simulink library "NeuroMuscularLibrary"  (R2019b)
settings: Solver=ode45  StartTime=0.0  StopTime=10.0  RelTol=1e-3  EnableMultiTasking=on
values from neighbouring files (symbols this model uses):
  a_18_19 = 116    [Prosthesis3R60Params.m]
  a_18_21 = 34    [Prosthesis3R60Params.m]
  a_2_3 = 18    [Prosthesis3R60Params.m]
  angle_offset = 0    [Prosthesis3R60Params.m]
  ankle_height = 0.08    [BodyMechParams.m]
  c = 0.05    [BodyMechParams.m]
  c_jointstop = 0.3 / (pi/180)    (= 17.1887338539)    [BodyMechParams.m]
  c_stance_comp_a0 = 885.0653    [Prosthesis3R60Params.m]
  c_stance_comp_a1 = 2.1443    [Prosthesis3R60Params.m]
  cg14 = 1/2*L14    (= 0.0475)    [Prosthesis3R60Params.m]
  cg25 = (5.45/11.05)*L25    (= 0.0379527149321)    [Prosthesis3R60Params.m]
  cg3 = (3.6/10.4)*L3    (= 0.0306346153846)    [Prosthesis3R60Params.m]
  d_fBall = 0.1    [BodyMechParams.m]
  d_fHeel = 0.05    [BodyMechParams.m]
  deltaLegAngleThr = 8*pi/180    (= 0.13962634016)    [CMGParams.m]
  DeltaThRef = 2e-3    (= 0.002)    [BodyMechParams.m]
  dt_visual = 0.001    [Prosthesis3R60Params.m]
  eref = 0.04    [BodyMechParams.m]
  Fmax = 4000    [MuscleEnergyTest.m]
  FmaxGLU = 1500    [BodyMechParams.m]
  footBallToAnkleDist = 0.16    [BodyMechParams.m]
  footBallToCenterDist = footLength/2    (= 0.1)    [BodyMechParams.m]
  footBallToHeelDist = footLength    (= 0.2)    [BodyMechParams.m]
  footCenterToCGDist = 0.14 - footBallToCenterDist    (= 0.04)    [BodyMechParams.m]
  footInertia = 0.005    [BodyMechParams.m]
  footLength = 0.2    [BodyMechParams.m]
  footMass = 1.25    [BodyMechParams.m]
  FT = 20    [MuscleEnergyTest.m]
  FT_GLU = 47.6    [BodyMechParams.m]
  g = 9.80665    [BodyMechParams.m]
  groundTheta = [atan(diff(groundZ)./diff(groundX)), 0]    [generateGround.m]
  groundZ = groundZ * stepSize/(largestStep+eps)    [generateGround.m]
  hatCenterToCGDist = 0.35 - hatHipToCenterDistLen    (= -0.05)    [BodyMechParams.m]
  hatHipToCenterDistLen = hatLength/2    (= 0.4)    [BodyMechParams.m]
  hatInertia = 3    [BodyMechParams.m]
  hatLeftHipToCenterDistWidth = .15    (= 0.15)    [BodyMechParams.m]
  hatLength = 0.8    [BodyMechParams.m]
  hatMass = 53.5    [BodyMechParams.m]
  hatThickness = 0.2    [BodyMechParams.m]
  hatWidth = 0.4    [BodyMechParams.m]
  J1011 = (4130)*1e-9    (= 4.13e-06)    [Prosthesis3R60Params.m]
  J1415 = (1.18*1e5)*1e-9    (= 0.000118)    [Prosthesis3R60Params.m]
  J18192021 = (6.86*1e4)*1e-9    (= 6.86e-05)    [Prosthesis3R60Params.m]
  J2526 = (3.59*1e4)*1e-9    (= 3.59e-05)    [Prosthesis3R60Params.m]
  J3467 = (25.96*1e4)*1e-9    (= 0.0002596)    [Prosthesis3R60Params.m]
  K = 5    [BodyMechParams.m]
  k_gn = k_gn/2    (= 39226.6)    [BodyMechParams.m]
  k_gt = k_gt/2    (= 39226.6)    [BodyMechParams.m]
  k_pressure = hatMass * g / DeltaThRef    (= 262327.8875)    [BodyMechParams.m]
  k_stance = 130000    [Prosthesis3R60Params.m]
  k_swing = 18750    [Prosthesis3R60Params.m]
  L0_stance = 0.08925    [Prosthesis3R60Params.m]
  L0_swing = 0.0896    [Prosthesis3R60Params.m]
  L10 = 7.9*1e-3    (= 0.0079)    [Prosthesis3R60Params.m]
  L11 = 3.3*1e-3    (= 0.0033)    [Prosthesis3R60Params.m]
  L14 = 95*1e-3    (= 0.095)    [Prosthesis3R60Params.m]
  L15 = 8.2*1e-3    (= 0.0082)    [Prosthesis3R60Params.m]
  L18 = 25.1*1e-3    (= 0.0251)    [Prosthesis3R60Params.m]
  L19 = 17.7*1e-3    (= 0.0177)    [Prosthesis3R60Params.m]
  L20 = 26*1e-3    (= 0.026)    [Prosthesis3R60Params.m]
  L21 = 1.7*1e-3    (= 0.0017)    [Prosthesis3R60Params.m]
  L25 = 76.95*1e-3    (= 0.07695)    [Prosthesis3R60Params.m]
  L26 = 2.8*1e-3    (= 0.0028)    [Prosthesis3R60Params.m]
  L3 = 88.5*1e-3    (= 0.0885)    [Prosthesis3R60Params.m]
  L4 = 1.7*1e-3    (= 0.0017)    [Prosthesis3R60Params.m]
  L6 = 40.25*1e-3    (= 0.04025)    [Prosthesis3R60Params.m]
  L7 = 14.9*1e-3    (= 0.0149)    [Prosthesis3R60Params.m]
  leg_l = [(thighLength - ankle_height/2) (shankLength - ankle_height/2)]    [BodyMechParams.m]
  legAngleSpeedMax = 10    [CMGParams.m]
  lopt = 0.055    [MuscleEnergyTest.m]
  loptBFSH = 0.12    [BodyMechParams.m]
  loptGAS = 0.05    [BodyMechParams.m]
  loptGLU = 0.11    [BodyMechParams.m]
  loptHAB = 0.09    [BodyMechParams.m]
  loptHAD = 0.10    (= 0.1)    [BodyMechParams.m]
  loptHAM = 0.10    (= 0.1)    [BodyMechParams.m]
  loptHFL = 0.11    [BodyMechParams.m]
  loptRF = 0.08    [BodyMechParams.m]
  loptSOL = 0.04    [BodyMechParams.m]
  loptTA = 0.06    [BodyMechParams.m]
  loptVAS = 0.08    [BodyMechParams.m]
  lslack = 0.245    [MuscleEnergyTest.m]
  lslackBFSH = 0.10    (= 0.1)    [BodyMechParams.m]
  lslackGAS = 0.40    (= 0.4)    [BodyMechParams.m]
  lslackGLU = 0.13    [BodyMechParams.m]
  lslackHAB = 0.07    [BodyMechParams.m]
  lslackHAD = 0.18    [BodyMechParams.m]
  lslackHAM = 0.31    [BodyMechParams.m]
  lslackHFL = 0.10    (= 0.1)    [BodyMechParams.m]
  lslackRF = 0.35    [BodyMechParams.m]
  lslackSOL = 0.26    [BodyMechParams.m]
  lslackTA = 0.24    [BodyMechParams.m]
  lslackVAS = 0.23    [BodyMechParams.m]
  m1011 = 49.5*1e-3    (= 0.0495)    [Prosthesis3R60Params.m]
  m1415 = 123.8*1e-3    (= 0.1238)    [Prosthesis3R60Params.m]
  m18192021 = 196.6*1e-3    (= 0.1966)    [Prosthesis3R60Params.m]
  m2526 = 58.3*1e-3    (= 0.0583)    [Prosthesis3R60Params.m]
  m3467 = 253.3*1e-3    (= 0.2533)    [Prosthesis3R60Params.m]
  mu_slide = 0.8    [BodyMechParams.m]
  mu_stick = 0.9    [BodyMechParams.m]
  N = 1.5    [BodyMechParams.m]    (also in cmaes.m = size(x,1); mergeCompareEnergyCosts.m = {S.name})
  phiKneeUpLimit = 5*pi/180    (= 0.0872664625997)    [BodyMechParams.m]
  phimaxGASa = (100-90)*pi/180    (= 0.174532925199)    [BodyMechParams.m]
  phimaxGASk = (180-140)*pi/180    (= 0.698131700798)    [BodyMechParams.m]
  phimaxRFk = (180-165)*pi/180    (= 0.261799387799)    [BodyMechParams.m]
  phimaxSOL = (100-90)*pi/180    (= 0.174532925199)    [BodyMechParams.m]
  phimaxTA = (80-90)*pi/180    (= -0.174532925199)    [BodyMechParams.m]
  phimaxVAS = (180-165)*pi/180    (= 0.261799387799)    [BodyMechParams.m]
  phirefBFSH = (180-160)*pi/180    (= 0.349065850399)    [BodyMechParams.m]
  phirefGASa = (80-90)*pi/180    (= -0.174532925199)    [BodyMechParams.m]
  phirefGASk = (180-165)*pi/180    (= 0.261799387799)    [BodyMechParams.m]
  phirefGLU = (120-180)*pi/180    (= -1.0471975512)    [BodyMechParams.m]
  phirefHAB = 10*pi/180    (= 0.174532925199)    [BodyMechParams.m]
  phirefHAD = 15*pi/180    (= 0.261799387799)    [BodyMechParams.m]
  phirefHAMh = (150-180)*pi/180    (= -0.523598775598)    [BodyMechParams.m]
  phirefHAMk = (180-180)*pi/180    (= 0)    [BodyMechParams.m]
  phirefHFL = (160-180)*pi/180    (= -0.349065850399)    [BodyMechParams.m]
  phirefRFh = (170-180)*pi/180    (= -0.174532925199)    [BodyMechParams.m]
  phirefRFk = (180-125)*pi/180    (= 0.959931088597)    [BodyMechParams.m]
  phirefSOL = (90-90)*pi/180    (= 0)    [BodyMechParams.m]
  ... (+64 more)
undefined symbols (not defined in the file or in its folder): ankleBackDriveGain, ankleCJointstop, ankleDgain, ankleFilterPID, ankleFilterSEA, ankleGearEff, ankleGearRatio, ankleIgain, ankleInitialAngle, ankleInputMass, ankleIntCoulomb, ankleIntDamping, ankleIntStatic, ankleParallelSpringDamping, ankleParallelSpringOffset, ankleParallelSpringStiffness, anklePgain, anklePlantarLimit, ankleSEADamping, ankleSEAStiffness, ankleTendonMass, ankleWMaxJointstop, D12_F, D12_S, D12_T, D12z_T, D13_F, D1G_F, D1G_HAT, D1G_S, D1G_T, D1Gy_F, DeltaS, DeltaSGLU, DeltaSHFL, dryFrictionDamping, dryFrictionStiffness, dryFrictionVelThresh, footMassp, FourBarL1, FourBarL3, GainDphiHATGLUst, GainDphiHATHABst, GainDphiHATHADst, GainDphiHATHFLst, GainFGASst, GainFGLUst, GainFHABst, GainFHAMst, GainFSOLst, GainFSOLTAst, GainFVASst, GainGAS, GainGLU, GainGLUswing, GainHAM, GainHAMHFL ... (+194)
libraries: sm_lib x332, nesl_utility x156, simulink x33, dspswit3 x30, $bdroot x19, simulink_extras x7
(part 8 of 15)

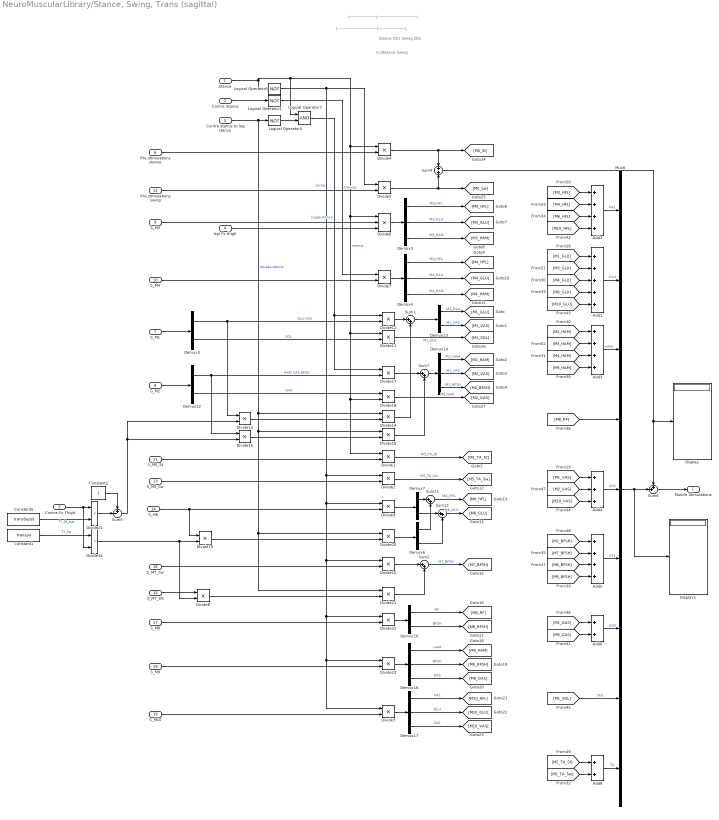
== system NeuroMuscularLibrary/Stance, Swing, Trans (sagittal) ==
  note: Stance DS1 Swing DS2
  note: FullStance Swing
  note: |------------------------------|--------------------|
  note: |--------------------|------------------------------|
  Stance : Inport
  Contra Stance : Inport  Port=2
  Contra stance to leg stance : Inport  Port=3
  Ispi Fx thigh : Inport  Port=4
  Contra Fx Thigh : Inport  Port=5
  Pre stimulations stance : Inport  Port=6
  S_M1 : Inport  Port=7
  S_M2 : Inport  Port=8
  S_M3 : Inport  Port=9
  S_M4 : Inport  Port=10
  S_M5_St : Inport  Port=11
  Pre stimulations swing : Inport  Port=12
  S_M5_Sw : Inport  Port=13
  S_M6 : Inport  Port=14
  S_M7_DS : Inport  Port=15
  S_M7_Sw : Inport  Port=16
  S_M8 : Inport  Port=17
  S_M9 : Inport  Port=18
  S_M10 : Inport  Port=19
  Add1 : Sum  Inputs=5
  Add2 : Sum  Inputs=4
  Add3 : Sum  Inputs=4
  Add4 : Sum  Inputs=3
  Add5 : Sum  Inputs=4
  Add6 : Sum  Inputs=2
  Add8 : Sum  Inputs=2
  Constant1 : Constant  Value=transsw
  Constant2 : Constant
  Constant5 : Constant  Value=transSupst
  Demux{6..7,10,13} (4 alike) : Demux  Outputs=2
  Demux12 : Demux  Outputs=[3 1]
  Demux{3..4,14,16..17} (5 alike) : Demux  Outputs=3
  Demux5 : Demux  Outputs=[2 1]
  Display : Display
  Display1 : Display
  Divide{1..5,7..24,34} (24 alike) : Product
  Divide6 : Product  Inputs=3
  Logical Operator1 : Logic  Operator=NOT  AllPortsSameDT=off  OutDataTypeStr=boolean
  Logical Operator5 : Logic  Operator=NOT  AllPortsSameDT=off  OutDataTypeStr=boolean
  Logical Operator6 : Logic  Operator=NOT  AllPortsSameDT=off  OutDataTypeStr=boolean
  Logical Operator7 : Logic  AllPortsSameDT=off  OutDataTypeStr=boolean
  Mux6 : Mux  Inputs=9
  Sum{1..2,7,11..12} (5 alike) : Sum  Inputs=|++  SaturateOnIntegerOverflow=on  InputSameDT=on  OutDataTypeStr=Inherit: Same as first input
  Sum4 : Sum  SaturateOnIntegerOverflow=on  InputSameDT=on  OutDataTypeStr=Inherit: Same as first input
  Sum5 : Sum  Inputs=+-|  SaturateOnIntegerOverflow=on  InputSameDT=on  OutDataTypeStr=Inherit: Same as first input
  Sum6 : Sum  Inputs=++|  SaturateOnIntegerOverflow=on  InputSameDT=on  OutDataTypeStr=Inherit: Same as first input
  Muscle Stimulations : Outport  OutputWhenDisabled=reset  InitialOutput=0
  wires:
  Stance/1 -> Logical Operator7/1, Divide4/1, Divide11/1, Divide18/2, Divide1/1, Divide6/1, Logical Operator6/1  "stance"
  Contra stance to leg stance/1 -> Logical Operator5/1, Divide14/1, Divide16/1, Divide20/1, Divide21/1  "double stance"
  Logical Operator5/1 -> Logical Operator7/2
  S_M4/1 -> Divide7/2
  Contra Stance/1 -> Logical Operator1/1
  Logical Operator1/1 -> Divide7/1  "Cswing"
  Constant5/1 -> Divide24/2  "Tr_St_sup"
  Divide24/1 -> Sum5/2
  Constant2/1 -> Sum5/1
  Contra Fx Thigh/1 -> Divide24/1, Divide34/2
  Demux4/1 -> [M4_HFL]  "M4_HFL"
  Add2/1 -> Mux6/1  "HFL"
  Add1/1 -> Mux6/2  "GLU"
  Demux4/2 -> [M4_GLU]  "M4_GLU"
  Add3/1 -> Mux6/3  "HAM"
  Demux4/3 -> [M4_HAM]  "M4_HAM"
  Add4/1 -> Mux6/5  "VAS"
  Add5/1 -> Mux6/6  "KFL"
  Add6/1 -> Mux6/7  "GAS"
  Add8/1 -> Mux6/9  "TA"
  Constant1/1 -> Divide34/1  "Tr_Sw"
  Divide7/1 -> Demux4/1
  Logical Operator7/1 -> Divide12/1, Divide17/1  "single stance"
  Divide34/1 -> Divide19/2, Divide8/2
  Logical Operator6/1 -> Divide5/1, Divide2/1, Divide9/1, Divide10/1, Divide3/1, Divide23/1, Divide22/1  "swing"
  Mux6/1 -> Display1/1, Sum6/2
  Sum6/1 -> Muscle Stimulations/1
  Sum4/1 -> Display/1, Sum6/1
  Pre stimulations swing/1 -> Divide5/2
  Pre stimulations stance/1 -> Divide4/2
  Divide5/1 -> [M0_Sw], Sum4/2
  Divide4/1 -> Sum4/1, [M0_St]
  S_M1/1 -> Demux5/1
  S_M2/1 -> Demux12/1
  Demux5/1 -> Divide12/2, Divide13/1  "GLU VAS"
  Demux5/2 -> Divide11/2  "SOL"
  Divide12/1 -> Sum1/1
  Divide13/1 -> Divide14/2
  Divide14/1 -> Sum1/2
  Divide16/1 -> Sum7/2
  Divide15/1 -> Divide16/2
  Sum1/1 -> Demux13/1
  Demux13/1 -> [M1_GLU]  "M1_GLU"
  Demux13/2 -> [M1_VAS]  "M1_VAS"
  Demux12/1 -> Divide17/2, Divide15/1  "HAM VAS BFSH"
  Divide17/1 -> Sum7/1
  Sum7/1 -> Demux14/1
  Demux14/1 -> [M2_HAM]  "M2_HAM"
  Demux14/2 -> [M2_VAS]  "M2_VAS"
  Demux14/3 -> [M2_BFSH]  "M2_BFSH"
  Demux12/2 -> Divide18/1  "GAS"
  Divide18/1 -> [M2_GAS]  "M2_GAS"
  S_M5_St/1 -> Divide1/2
  Divide1/1 -> [M5_TA_St]  "M5_TA_St"
  Divide11/1 -> [M1_SOL]  "M1_SOL"
  S_M3/1 -> Divide6/2
  Ispi Fx thigh/1 -> Divide6/3
  Divide6/1 -> Demux3/1
  Demux3/1 -> [M3_HFL]  "M3_HFL"
  Demux3/2 -> [M3_GLU]  "M3_GLU"
  Demux3/3 -> [M3_HAM]  "M3_HAM"
  S_M5_Sw/1 -> Divide2/2
  Divide2/1 -> [M5_TA_Sw]  "M5_TA_Sw"
  S_M6/1 -> Divide9/2, Divide19/1
  Divide9/1 -> Demux7/1
  Demux7/2 -> Sum12/1
  Divide20/1 -> Demux6/1
  Demux6/1 -> Sum11/2
  Demux6/2 -> Sum12/2
  Demux7/1 -> Sum11/1
  Divide19/1 -> Divide20/2
  Sum11/1 -> [M6_HFL]  "M6_HFL"
  Sum12/1 -> [M6_GLU]  "M6_GLU"
  Divide10/1 -> Sum2/1
  Divide21/1 -> Sum2/2
  Sum5/1 -> Divide13/2, Divide15/2
  S_M7_Sw/1 -> Divide10/2
  Divide8/1 -> Divide21/2
  S_M7_DS/1 -> Divide8/1
  Sum2/1 -> [M7_BFSH]  "M7_BFSH"
  S_M8/1 -> Divide22/2
  Divide22/1 -> Demux10/1
  S_M9/1 -> Divide23/2
  Divide23/1 -> Demux16/1
  S_M10/1 -> Divide3/2
  Divide3/1 -> Demux17/1
  Demux10/2 -> [M8_BFSH]  "BFSH"
  Demux10/1 -> [M8_RF]  "RF"
  Demux16/1 -> [M9_HAM]  "HAM"
  Demux16/2 -> [M9_BFSH]  "BFSH"
  Demux16/3 -> [M9_GAS]  "GAS"
  Demux17/1 -> [M10_HFL]  "HFL"
  Demux17/2 -> [M10_GLU]  "GLU"
  Demux17/3 -> [M10_VAS]  "VAS"
  [M1_GLU] -> Add1/1
  [M3_GLU] -> Add1/2
  [M4_GLU] -> Add1/3
  [M6_GLU] -> Add1/4
  [M10_GLU] -> Add1/5
  [M1_VAS] -> Add4/1
  [M2_HAM] -> Add3/1
  [M2_VAS] -> Add4/2
  [M2_BFSH] -> Add5/1
  [M2_GAS] -> Add6/1
  [M3_HFL] -> Add2/1
  [M3_HAM] -> Add3/2
  [M4_HFL] -> Add2/2
  [M4_HAM] -> Add3/3
  [M5_TA_St] -> Add8/1
  [M5_TA_Sw] -> Add8/2
  [M6_HFL] -> Add2/3
  [M7_BFSH] -> Add5/2
  [M9_BFSH] -> Add5/4
  [M8_BFSH] -> Add5/3
  [M8_RF] -> Mux6/4
  [M9_HAM] -> Add3/4
  [M9_GAS] -> Add6/2
  [M10_HFL] -> Add2/4
  [M10_VAS] -> Add4/3
  [M1_SOL] -> Mux6/8  "SOL"

== system NeuroMuscularLibrary/Stimulation Mixing ==
  Stance Stim : Inport
  dxThigh : Inport  Port=2
  Stance? : Inport  Port=3
  ContraLegLeading? : Inport  Port=4
  Swing Stim : Inport  Port=5
  Constant : Constant
  FB Gain1 : Gain  Gain=1/DeltaThRef  SaturateOnIntegerOverflow=on  OutDataTypeStr=Inherit: Same as input  ParamDataTypeStr=Inherit: Same as input
  Logical Operator : Logic  Operator=NOT  AllPortsSameDT=off  OutDataTypeStr=boolean
  Logical Operator1 : Logic  Operator=NOT  AllPortsSameDT=off  OutDataTypeStr=boolean
  Product{,1..3} (4 alike) : Product
  Product4 : Product  Inputs=3
  Saturation17 : Saturate  UpperLimit=1  LowerLimit=0.01  ZeroCross=off
  Saturation2 : Saturate  UpperLimit=1  LowerLimit=0  ZeroCross=off
  Sum : Sum  Inputs=+|+
  Sum1 : Sum  Inputs=-+|
  Sum3 : Sum  Inputs=+++
  stimulation : Outport  OutputWhenDisabled=reset
  wires:
  dxThigh/1 -> FB Gain1/1
  Stance Stim/1 -> Product4/1, Product/1
  FB Gain1/1 -> Saturation2/1
  Saturation2/1 -> Product/2, Sum1/1
  Swing Stim/1 -> Product3/1, Product1/2
  Constant/1 -> Sum1/2
  Sum1/1 -> Product1/1
  Product1/1 -> Sum/2
  Product/1 -> Sum/1
  Logical Operator/1 -> Product4/3
  Stance?/1 -> Logical Operator1/1, Product4/2
  Sum/1 -> Product2/1
  Product2/1 -> Sum3/2  "Mixed Stimulation"
  Sum3/1 -> Saturation17/1
  Saturation17/1 -> stimulation/1
  Product4/1 -> Sum3/1  "Stance Stimulation Only"
  Logical Operator1/1 -> Product3/2
  Product3/1 -> Sum3/3  "Swing Stimulation Only"
  ContraLegLeading?/1 -> Product2/2, Logical Operator/1

== system NeuroMuscularLibrary/Subsystem ==
  Thigh dx : Inport

== system NeuroMuscularLibrary/Swing Hip & Ankles ==
  note: Stimulation
  note: Torques
  note: Hip Torque
  note: GLU Control
  note: GAS Control
  note: TA Control
  note: VAS Control
  note: SOL Control
  note: HAM Control
  note: HFL Control
  Muscle Torques : Inport
  LceTA : Inport  Port=2
  FmHAM : Inport  Port=3
  FmGLU : Inport  Port=4
  LceHFL : Inport  Port=5
  LceHAM : Inport  Port=6
  phiANDdphiHAT : Inport  Port=7
  " 3" : Gain  Gain=GainTA
  Add3 : Sum
  Add4 : Sum  Inputs=++-+
  Add7 : Sum
  Add8 : Sum
  Constant1 : Constant  Value=PreStimGAS
  Constant2 : Constant  Value=PreStimVAS
  Constant4 : Constant  Value=PreStimTA
  Constant6 : Constant  Value=PreStimSOL
  Count Extend : dspswit3/Counter  Direction=Up  CountEvent=Rising edge  CounterSize=16 bits  MaxCount=255  InitialCount=0  Output=Count  HitValue=32  ResetInput=off  SamplesPerFrame=1  Ts=1  CntDtype=double  HitDtype=Logical
  Count Flex : dspswit3/Counter  Direction=Up  CountEvent=Rising edge  CounterSize=16 bits  MaxCount=255  InitialCount=0  Output=Count  HitValue=32  ResetInput=off  SamplesPerFrame=1  Ts=1  CntDtype=double  HitDtype=Logical
  Count Hold : dspswit3/Counter  Direction=Up  CountEvent=Rising edge  CounterSize=16 bits  MaxCount=255  InitialCount=0  Output=Count  HitValue=32  ResetInput=off  SamplesPerFrame=1  Ts=1  CntDtype=double  HitDtype=Logical
  Count Stancea : dspswit3/Counter  Direction=Up  CountEvent=Rising edge  CounterSize=16 bits  MaxCount=255  InitialCount=0  Output=Count  HitValue=32  ResetInput=off  SamplesPerFrame=1  Ts=1  CntDtype=double  HitDtype=Logical
  Count Stop : dspswit3/Counter  Direction=Up  CountEvent=Rising edge  CounterSize=16 bits  MaxCount=255  InitialCount=0  Output=Count  HitValue=32  ResetInput=off  SamplesPerFrame=1  Ts=1  CntDtype=double  HitDtype=Logical
  Demux : Demux  Outputs=3
  Demux2 : Demux  Outputs=2
  FB Gain1 : Gain  Gain=GainHAM  SaturateOnIntegerOverflow=on  OutDataTypeStr=Inherit: Same as input  ParamDataTypeStr=Inherit: Same as input
  FB Gain11 : Gain  Gain=Klean  SaturateOnIntegerOverflow=on  OutDataTypeStr=Inherit: Same as input  ParamDataTypeStr=Inherit: Same as input
  FB Gain2 : Gain  Gain=GainHFL  SaturateOnIntegerOverflow=on  OutDataTypeStr=Inherit: Same as input  ParamDataTypeStr=Inherit: Same as input
  FB Gain4 : Gain  Gain=GainHAMHFL  SaturateOnIntegerOverflow=on  OutDataTypeStr=Inherit: Same as input  ParamDataTypeStr=Inherit: Same as input
  FB Gain5 : Gain  Gain=GainGLU  SaturateOnIntegerOverflow=on  OutDataTypeStr=Inherit: Same as input  ParamDataTypeStr=Inherit: Same as input
  Multiply : Gain
  Multiply1 : Gain
  Multiply2 : Gain
  Mux1 : Mux  Inputs=7
  Mux2 : Mux  Inputs=3
  Mux3 : Mux  Inputs=5
  Mux4 : Mux  Inputs=3
  Stimulation Bias4 : Constant  Value=PreStimHFL
  Stimulation Bias5 : Constant  Value=PreStimHAM
  Stimulation Bias6 : Constant  Value=phiHATref
  Stimulation Bias8 : Constant  Value=PreStimGLU
  Sum9 : Sum  Inputs=|+-  SaturateOnIntegerOverflow=on  InputSameDT=on  OutDataTypeStr=Inherit: Same as first input
  Terminator : Terminator
  ideal ankle torque{,1..7} (8 alike) : Constant  Value=0
  Stimulation : Outport
  Swing Muscle Torques : Outport  Port=2
  Swing Ideal Torques : Outport  Port=3
  Swing State Counts : Outport  Port=4
  wires:
  Demux/2 -> Mux4/2
  Demux/3 -> Mux4/3
  Mux4/1 -> Swing Muscle Torques/1
  Constant6/1 -> Mux1/1
  Add3/1 -> Mux1/2
  Add8/1 -> Mux1/6
  Add4/1 -> Mux1/7
  Add7/1 -> Mux1/5
  ideal ankle torque3/1 -> Count Stancea/1
  ideal ankle torque6/1 -> Count Stop/1
  Count Flex/1 -> Mux3/2
  ideal ankle torque1/1 -> Mux2/2
  ideal ankle torque2/1 -> Mux2/1
  ideal ankle torque5/1 -> Count Hold/1
  Count Hold/1 -> Mux3/3
  ideal ankle torque/1 -> Mux2/3
  Mux3/1 -> Swing State Counts/1
  Count Stancea/1 -> Mux3/1
  ideal ankle torque4/1 -> Count Flex/1
  ideal ankle torque7/1 -> Count Extend/1
  Mux2/1 -> Swing Ideal Torques/1
  Count Extend/1 -> Mux3/5
  Mux1/1 -> Stimulation/1
  FmHAM/1 -> FB Gain1/1
  " 3"/1 -> Add3/2
  phiANDdphiHAT/1 -> Demux2/1
  LceHFL/1 -> FB Gain2/1
  Stimulation Bias8/1 -> Multiply/1
  Stimulation Bias5/1 -> Multiply2/1
  Constant2/1 -> Mux1/4
  Sum9/1 -> FB Gain11/1
  FB Gain5/1 -> Add8/2
  Demux/1 -> Mux4/1
  FmGLU/1 -> FB Gain5/1
  Demux2/1 -> Sum9/1  "phiHAT"
  Count Stop/1 -> Mux3/4
  LceTA/1 -> " 3"/1
  Demux2/2 -> Terminator/1  "dphiHat"
  Muscle Torques/1 -> Demux/1
  FB Gain11/1 -> Add4/4
  Stimulation Bias6/1 -> Sum9/2
  LceHAM/1 -> FB Gain4/1
  FB Gain2/1 -> Add4/2
  Stimulation Bias4/1 -> Multiply1/1
  FB Gain1/1 -> Add7/2
  FB Gain4/1 -> Add4/3
  Constant1/1 -> Mux1/3
  Multiply/1 -> Add8/1
  Multiply1/1 -> Add4/1
  Multiply2/1 -> Add7/1
  Constant4/1 -> Add3/1

== system NeuroMuscularLibrary/Swing Phase ==
  note: Stimulation
  note: SOL Control
  note: GAS Control
  note: TA Control
  note: VAS Control
  note: HAM Control
  note: GLU Control
  note: HFL Control
  note: Torques
  note: Hip Torque
  note: only ankle muscle torque
  Muscle Torques : Inport
  LceTA : Inport  Port=2
  Leg Angle : Inport  Port=3
  Leg Length : Inport  Port=4
  Stance? : Inport  Port=5
  contraStance? : Inport  Port=6
  Knee Speed : Inport  Port=7
  Target Leg Angle : Inport  Port=8
  " 1" : Gain  Gain=hipPGain
  " 2" : Gain  Gain=hipDGain
  " 3" : Gain  Gain=GainTA
  " 4" : Gain  Gain=2
  " 5" : Gain  Gain=0
  " 6" : Gain  Gain=0
  Add : Sum  Inputs=+++
  Add1 : Sum  Inputs=+-+
  Add3 : Sum
  Chart : Stateflow chart  TreatAsAtomicUnit=on
  Constant{1..3,5..7} (6 alike) : Constant  Value=0
  Constant4 : Constant  Value=PreStimTA
  Count Extend : dspswit3/Counter  Direction=Up  CountEvent=Rising edge  CounterSize=16 bits  MaxCount=255  InitialCount=0  Output=Count  HitValue=32  ResetInput=off  SamplesPerFrame=1  Ts=1  CntDtype=double  HitDtype=Logical
  Count Flex : dspswit3/Counter  Direction=Up  CountEvent=Rising edge  CounterSize=16 bits  MaxCount=255  InitialCount=0  Output=Count  HitValue=32  ResetInput=off  SamplesPerFrame=1  Ts=1  CntDtype=double  HitDtype=Logical
  Count Hold : dspswit3/Counter  Direction=Up  CountEvent=Rising edge  CounterSize=16 bits  MaxCount=255  InitialCount=0  Output=Count  HitValue=32  ResetInput=off  SamplesPerFrame=1  Ts=1  CntDtype=double  HitDtype=Logical
  Count Stancea : dspswit3/Counter  Direction=Up  CountEvent=Rising edge  CounterSize=16 bits  MaxCount=255  InitialCount=0  Output=Count  HitValue=32  ResetInput=off  SamplesPerFrame=1  Ts=1  CntDtype=double  HitDtype=Logical
  Count Stop : dspswit3/Counter  Direction=Up  CountEvent=Rising edge  CounterSize=16 bits  MaxCount=255  InitialCount=0  Output=Count  HitValue=32  ResetInput=off  SamplesPerFrame=1  Ts=1  CntDtype=double  HitDtype=Logical
  Demux : Demux  Outputs=3
  Filtered Derivative : Subsystem
  Knee Flex : Subsystem  TreatAsAtomicUnit=on
  Knee Hold : Subsystem  TreatAsAtomicUnit=on
  Knee Stop : Subsystem  TreatAsAtomicUnit=on
  Mux1 : Mux  Inputs=7
  Mux2 : Mux  Inputs=3
  Mux3 : Mux  Inputs=5
  Mux4 : Mux  Inputs=3
  Sum : Sum  Inputs=|+-
  Wait 100 ms to enable : Subsystem
  Zero-Order Hold : ZeroOrderHold  SampleTime=.01
  ideal ankle torque : Constant  Value=0
  Stimulation : Outport
  Swing Ideal Torques : Outport  Port=2
  Swing Muscle Torques : Outport  Port=3
  Swing State Counts : Outport  Port=4
  wires:
  Demux/3 -> Mux4/3
  " 6"/1 -> Mux4/2
  " 5"/1 -> Mux4/1
  Demux/2 -> " 6"/1
  Demux/1 -> " 5"/1
  Muscle Torques/1 -> Demux/1
  Mux4/1 -> Swing Muscle Torques/1
  Mux2/1 -> Swing Ideal Torques/1
  ideal ankle torque/1 -> Mux2/3
  Zero-Order Hold/1 -> Count Stancea/1
  Count Stancea/1 -> Mux3/1
  Mux3/1 -> Swing State Counts/1
  Count Flex/1 -> Mux3/2
  Count Hold/1 -> Mux3/3
  Count Stop/1 -> Mux3/4
  Count Extend/1 -> Mux3/5
  Add1/1 -> Mux2/1  "Hip Torque"
  Leg Length/1 -> Knee Stop/4(Leg Length), Chart/6(legLength)
  contraStance?/1 -> Chart/2(contraStance)
  Stance?/1 -> Chart/1(Stance), Zero-Order Hold/1
  Chart/4(extend) -> Knee Stop/5(Extend?), Count Extend/1
  Chart/3(stop) -> Knee Stop/Enable, Count Stop/1
  Chart/2(hold) -> Knee Hold/Enable, Count Hold/1
  Chart/1(flex) -> Count Flex/1, Knee Flex/Enable
  " 4"/1 -> Add1/3
  Add/1 -> Mux2/2
  Knee Stop/1(tau) -> Add/3, " 4"/1
  Knee Flex/1(tau) -> Add/1
  Knee Hold/1(tau) -> Add/2
  Knee Speed/1 -> Knee Hold/4(kneeSpeed)
  Constant4/1 -> Add3/1
  " 3"/1 -> Add3/2
  LceTA/1 -> " 3"/1
  Add3/1 -> Mux1/2
  Constant6/1 -> Mux1/1
  Constant5/1 -> Mux1/3
  Constant1/1 -> Mux1/4
  Constant2/1 -> Mux1/5
  Constant3/1 -> Mux1/6
  Constant7/1 -> Mux1/7
  Mux1/1 -> Stimulation/1
  Leg Angle/1 -> Sum/2, Knee Hold/2(legAngle), Knee Stop/2(legAngle), Chart/3(legAngle), Filtered Derivative/1(In1)  "Leg Angle"
  Sum/1 -> " 1"/1
  " 1"/1 -> Add1/1
  " 2"/1 -> Add1/2
  Target Leg Angle/1 -> Knee Hold/3(legAngleTgt), Knee Stop/3(legAngleTgt), Chart/5(legAngleTgt), Sum/1
  Filtered Derivative/1(Out1) -> Wait 100 ms to enable/1(In1)
  Wait 100 ms to enable/1(Out1) -> " 2"/1, Knee Flex/1(LegAngleSpeed), Knee Stop/1(legAngleSpeed), Knee Hold/1(legAngleSpeed), Chart/4(legAngleSpeed)

== system NeuroMuscularLibrary/Swing Phase (coronal) ==
  note: Swing Phase Control
  note: M6: swing hip
  Target Angle Coronal : Inport
  LceHAD : Inport  Port=2
  LceHAB : Inport  Port=3
  Enable : EnablePort  StatesWhenEnabling=reset  ZeroCross=off
  " 1" : Gain  Gain=R_Sw_a2lopt_HAB
  " 2" : Gain  Gain=R_Sw_a2lopt_HAD
  " 3" : Gain  Gain=GainLHABsw
  " 4" : Gain  Gain=GainLHADsw
  Constant1 : Constant
  Constant12 : Constant  Value=PreStimHADsw
  Constant15 : Constant  Value=PreStimHABsw
  Constant2 : Constant  Value=R_Sw_aRef_HAB
  Constant3 : Constant  Value=R_Sw_aRef_HAD
  Constant5 : Constant
  Mux : Mux  Inputs=2
  Mux1 : Mux  Inputs=2
  Sum1 : Sum  Inputs=-+|  SaturateOnIntegerOverflow=on  InputSameDT=on  OutDataTypeStr=Inherit: Same as first input
  Sum10 : Sum  Inputs=++|  SaturateOnIntegerOverflow=on  InputSameDT=on  OutDataTypeStr=Inherit: Same as first input
  Sum13 : Sum  Inputs=|-+  SaturateOnIntegerOverflow=on  InputSameDT=on  OutDataTypeStr=Inherit: Same as first input
  Sum2 : Sum  Inputs=-+|  SaturateOnIntegerOverflow=on  InputSameDT=on  OutDataTypeStr=Inherit: Same as first input
  Sum3 : Sum  Inputs=+-|  SaturateOnIntegerOverflow=on  InputSameDT=on  OutDataTypeStr=Inherit: Same as first input
  Sum4 : Sum  Inputs=+-|  SaturateOnIntegerOverflow=on  InputSameDT=on  OutDataTypeStr=Inherit: Same as first input
  positive half1 : Saturate  UpperLimit=inf  LowerLimit=0  ZeroCross=off
  positive half2 : Saturate  UpperLimit=inf  LowerLimit=0  ZeroCross=off
  S_0_Sw : Outport  OutputWhenDisabled=reset  InitialOutput=0
  S_M6 [HAB HAD] : Outport  Port=2  OutputWhenDisabled=reset  InitialOutput=0
  wires:
  Mux/1 -> S_0_Sw/1
  Constant5/1 -> Sum10/1
  Sum13/1 -> " 1"/1
  " 1"/1 -> Sum10/2
  Sum10/1 -> Sum1/1  "lceOffHAB"
  Sum1/1 -> positive half2/1
  positive half2/1 -> " 3"/1
  Constant1/1 -> Sum3/1
  Target Angle Coronal/1 -> Sum13/2, Sum4/1
  Sum4/1 -> " 2"/1
  " 2"/1 -> Sum3/2
  Sum3/1 -> Sum2/1  "lceOffHAD"
  Sum2/1 -> positive half1/1
  positive half1/1 -> " 4"/1
  LceHAB/1 -> Sum1/2
  LceHAD/1 -> Sum2/2
  " 3"/1 -> Mux1/1  "HAB"
  " 4"/1 -> Mux1/2  "HAD"
  Mux1/1 -> S_M6 [HAB HAD]/1
  Constant15/1 -> Mux/1
  Constant12/1 -> Mux/2
  Constant2/1 -> Sum13/1
  Constant3/1 -> Sum4/2

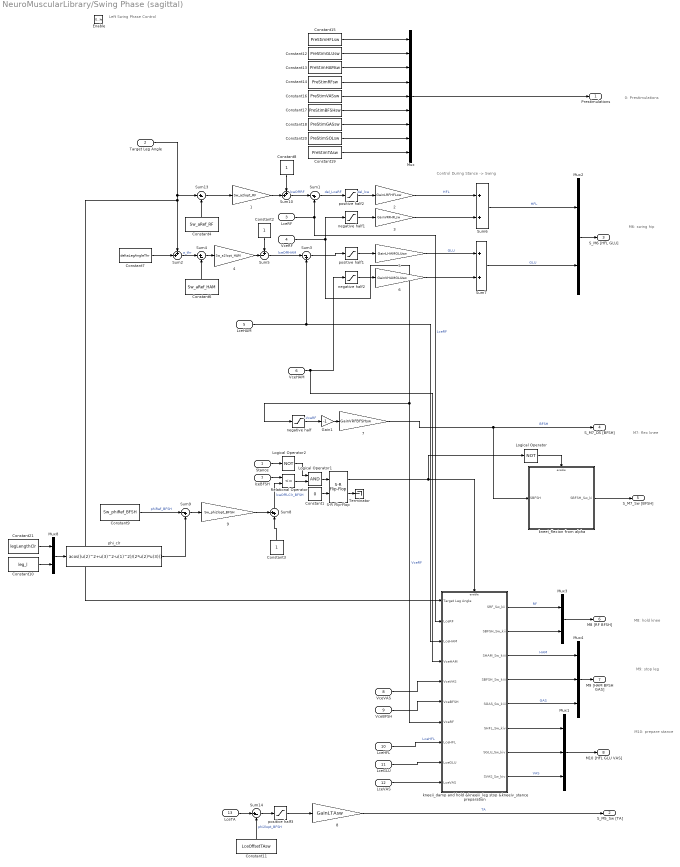
== system NeuroMuscularLibrary/Swing Phase (sagittal) ==
  note: Left Swing Phase Control
  note: Control During Stance -> Swing
  note: 0: Prestimulations
  note: M6: swing hip
  note: M7: flex knee
  note: M8: hold knee
  note: M9: stop leg
  note: M10: prepare stance
  Stance : Inport
  "Target Leg Angle " : Inport  Port=2
  LceRF : Inport  Port=3
  VceRF : Inport  Port=4
  LceHAM : Inport  Port=5
  VceHAM : Inport  Port=6
  lceBFSH : Inport  Port=7
  VceVAS : Inport  Port=8
  VceBFSH : Inport  Port=9
  LceHFL : Inport  Port=10
  LceGLU : Inport  Port=11
  LceVAS : Inport  Port=12
  LceTA : Inport  Port=13
  Enable : EnablePort  StatesWhenEnabling=reset  ZeroCross=off
  " 1" : Gain  Gain=Sw_a2lopt_RF
  " 2" : Gain  Gain=GainLRFHFLsw
  " 3" : Gain  Gain=GainVRFHFLsw
  " 4" : Gain  Gain=Sw_a2lopt_HAM
  " 5" : Gain  Gain=GainLHAMGLUsw
  " 6" : Gain  Gain=GainVHAMGLUsw
  " 7" : Gain  Gain=GainVRFBFSHsw
  " 8" : Gain  Gain=GainLTAsw
  " 9" : Gain  Gain=Sw_phi2lopt_BFSH
  Constant1 : Constant  Value=0  OutDataTypeStr=boolean
  Constant10 : Constant  Value=leg_l
  Constant11 : Constant  Value=LceOffsetTAsw
  Constant12 : Constant  Value=PreStimGLUsw
  Constant13 : Constant  Value=PreStimHAMsw
  Constant14 : Constant  Value=PreStimRFsw
  Constant15 : Constant  Value=PreStimHFLsw
  Constant16 : Constant  Value=PreStimVASsw
  Constant17 : Constant  Value=PreStimBFSHsw
  Constant18 : Constant  Value=PreStimGASsw
  Constant19 : Constant  Value=PreStimTAsw
  Constant2 : Constant
  Constant20 : Constant  Value=PreStimSOLsw
  Constant21 : Constant  Value=legLengthClr
  Constant3 : Constant
  Constant4 : Constant  Value=Sw_aRef_RF
  Constant6 : Constant  Value=Sw_aRef_HAM
  Constant7 : Constant  Value=deltaLegAngleThr
  Constant8 : Constant
  Constant9 : Constant  Value=Sw_phiRef_BFSH
  Gain1 : Gain  Gain=-1
  Logical Operator : Logic  Operator=NOT  AllPortsSameDT=off  OutDataTypeStr=boolean
  Logical Operator1 : Logic  AllPortsSameDT=off  OutDataTypeStr=boolean
  Logical Operator2 : Logic  Operator=NOT  AllPortsSameDT=off  OutDataTypeStr=boolean
  Mux : Mux  Inputs=9
  Mux1 : Mux  Inputs=3
  Mux2 : Mux  Inputs=2
  Mux3 : Mux  Inputs=2
  Mux4 : Mux  Inputs=3
  Mux8 : Mux  Inputs=2
  Relational Operator : RelationalOperator  Operator=<=  OutDataTypeStr=boolean  ZeroCross=off  RndMeth=Nearest
  S-R Flip-Flop : simulink_extras/Flip Flops/S-R Flip-Flop  initial_condition=0
  Sum1 : Sum  Inputs=|-+  SaturateOnIntegerOverflow=on  InputSameDT=on  OutDataTypeStr=Inherit: Same as first input
  Sum10 : Sum  Inputs=++|  SaturateOnIntegerOverflow=on  InputSameDT=on  OutDataTypeStr=Inherit: Same as first input
  Sum13 : Sum  Inputs=|+-  SaturateOnIntegerOverflow=on  InputSameDT=on  OutDataTypeStr=Inherit: Same as first input
  Sum14 : Sum  Inputs=|+-  SaturateOnIntegerOverflow=on  InputSameDT=on  OutDataTypeStr=Inherit: Same as first input
  Sum2 : Sum  Inputs=++|  SaturateOnIntegerOverflow=on  InputSameDT=on  OutDataTypeStr=Inherit: Same as first input
  Sum3 : Sum  Inputs=|-+  SaturateOnIntegerOverflow=on  InputSameDT=on  OutDataTypeStr=Inherit: Same as first input
  Sum4 : Sum  Inputs=|+-  SaturateOnIntegerOverflow=on  InputSameDT=on  OutDataTypeStr=Inherit: Same as first input
  Sum5 : Sum  Inputs=+-|  SaturateOnIntegerOverflow=on  InputSameDT=on  OutDataTypeStr=Inherit: Same as first input
  Sum6 : Sum  SaturateOnIntegerOverflow=on  InputSameDT=on  OutDataTypeStr=Inherit: Same as first input
  Sum7 : Sum  SaturateOnIntegerOverflow=on  InputSameDT=on  OutDataTypeStr=Inherit: Same as first input
  Sum8 : Sum  Inputs=++|  SaturateOnIntegerOverflow=on  InputSameDT=on  OutDataTypeStr=Inherit: Same as first input
  Sum9 : Sum  Inputs=|-+  SaturateOnIntegerOverflow=on  InputSameDT=on  OutDataTypeStr=Inherit: Same as first input
  Terminator : Terminator
  kneei_flexion from alpha : Subsystem  TreatAsAtomicUnit=on
  kneeii_damp and hold &kneeiii_leg stop &kneeiv_stance preparation : Subsystem  TreatAsAtomicUnit=on
  negative half : Saturate  UpperLimit=0  LowerLimit=-inf  ZeroCross=off
  negative half1 : Saturate  UpperLimit=0  LowerLimit=-inf  ZeroCross=off
  negative half2 : Saturate  UpperLimit=0  LowerLimit=-inf  ZeroCross=off
  phi_clr : Fcn  Expr=acos((u(2)^2+u(3)^2-u(1)^2)/(2*u(2)*u(3)))
  positive half1 : Saturate  UpperLimit=inf  LowerLimit=0  ZeroCross=off
  positive half2 : Saturate  UpperLimit=inf  LowerLimit=0  ZeroCross=off
  positive half3 : Saturate  UpperLimit=inf  LowerLimit=0  ZeroCross=off
  Prestimulations : Outport  OutputWhenDisabled=reset  InitialOutput=0
  S_M5_Sw [TA] : Outport  Port=2  OutputWhenDisabled=reset  InitialOutput=0
  S_M6 [HFL GLU] : Outport  Port=3  OutputWhenDisabled=reset  InitialOutput=0
  S_M7_DS [BFSH] : Outport  Port=4  OutputWhenDisabled=reset  InitialOutput=0
  S_M7_Sw [BFSH] : Outport  Port=5  OutputWhenDisabled=reset  InitialOutput=0
  M8 [RF BFSH] : Outport  Port=6  OutputWhenDisabled=reset  InitialOutput=0
  M9 [HAM BFSH GAS] : Outport  Port=7  OutputWhenDisabled=reset  InitialOutput=0
  M10 [HFL GLU VAS] : Outport  Port=8  OutputWhenDisabled=reset  InitialOutput=0
  wires:
  "Target Leg Angle "/1 -> kneeii_damp and hold &kneeiii_leg stop &kneeiv_stance preparation/1(Target Leg Angle), Sum2/1, Sum13/1
  Sum13/1 -> " 1"/1
  " 1"/1 -> Sum10/2
  Sum1/1 -> positive half2/1  "del_LceRF"
  positive half2/1 -> " 2"/1  "del_lce"
  Sum2/1 -> Sum4/1  "a_thr"
  Constant2/1 -> Sum5/1
  " 4"/1 -> Sum5/2
  Sum3/1 -> positive half1/1
  positive half1/1 -> " 5"/1
  Sum5/1 -> Sum3/1  "lceOffHAM"
  LceHAM/1 -> Sum3/2, kneeii_damp and hold &kneeiii_leg stop &kneeiv_stance preparation/3(LceHAM)
  Gain1/1 -> " 7"/1
  negative half/1 -> Gain1/1  "-VceRF"
  " 7"/1 -> kneei_flexion from alpha/1(SBFSH), S_M7_DS [BFSH]/1  "BFSH"
  Constant1/1 -> S-R Flip-Flop/2
  S-R Flip-Flop/2 -> Terminator/1
  S-R Flip-Flop/1 -> Logical Operator/1, kneeii_damp and hold &kneeiii_leg stop &kneeiv_stance preparation/Enable
  Logical Operator/1 -> kneei_flexion from alpha/Enable
  lceBFSH/1 -> Relational Operator/1
  Mux8/1 -> phi_clr/1
  Constant21/1 -> Mux8/1
  Constant10/1 -> Mux8/2
  Sum9/1 -> " 9"/1
  Constant9/1 -> Sum9/1  "phiRef_BFSH"
  phi_clr/1 -> Sum9/2
  Constant3/1 -> Sum8/2
  " 9"/1 -> Sum8/1
  Sum8/1 -> Relational Operator/2  "lceOffLClr_BFSH"
  VceBFSH/1 -> kneeii_damp and hold &kneeiii_leg stop &kneeiv_stance preparation/6(VceBFSH)
  LceHFL/1 -> kneeii_damp and hold &kneeiii_leg stop &kneeiv_stance preparation/8(LceHFL)  "LceHFL"
  LceGLU/1 -> kneeii_damp and hold &kneeiii_leg stop &kneeiv_stance preparation/9(LceGLU)
  LceVAS/1 -> kneeii_damp and hold &kneeiii_leg stop &kneeiv_stance preparation/10(LceVAS)
  kneeii_damp and hold &kneeiii_leg stop &kneeiv_stance preparation/6(SHFL_Sw_kiv) -> Mux1/1
  kneeii_damp and hold &kneeiii_leg stop &kneeiv_stance preparation/7(SGLU_Sw_kiv) -> Mux1/2
  kneei_flexion from alpha/1(SBFSH_Sw_ki) -> S_M7_Sw [BFSH]/1
  kneeii_damp and hold &kneeiii_leg stop &kneeiv_stance preparation/2(SBFSH_Sw_kii) -> Mux3/2
  kneeii_damp and hold &kneeiii_leg stop &kneeiv_stance preparation/4(SBFSH_Sw_kiii) -> Mux4/2
  Sum14/1 -> positive half3/1
  LceTA/1 -> Sum14/1
  positive half3/1 -> " 8"/1
  Logical Operator1/1 -> S-R Flip-Flop/1
  Relational Operator/1 -> Logical Operator1/2
  Stance/1 -> Logical Operator2/1
  Logical Operator2/1 -> Logical Operator1/1
  kneeii_damp and hold &kneeiii_leg stop &kneeiv_stance preparation/3(SHAM_Sw_kiii) -> Mux4/1  "HAM"
  kneeii_damp and hold &kneeiii_leg stop &kneeiv_stance preparation/1(SRF_Sw_kii) -> Mux3/1  "RF"
  kneeii_damp and hold &kneeiii_leg stop &kneeiv_stance preparation/8(SVAS_Sw_kiv) -> Mux1/3  "VAS"
  " 8"/1 -> S_M5_Sw [TA]/1  "TA"
  kneeii_damp and hold &kneeiii_leg stop &kneeiv_stance preparation/5(SGAS_Sw_kiii) -> Mux4/3  "GAS"
  Mux2/1 -> S_M6 [HFL GLU]/1
  Mux3/1 -> M8 [RF BFSH]/1
  Mux4/1 -> M9 [HAM BFSH GAS]/1
  Mux1/1 -> M10 [HFL GLU VAS]/1
  LceRF/1 -> kneeii_damp and hold &kneeiii_leg stop &kneeiv_stance preparation/2(LceRF), Sum1/2  "LceRF"
  VceVAS/1 -> kneeii_damp and hold &kneeiii_leg stop &kneeiv_stance preparation/5(VceVAS)
  VceRF/1 -> kneeii_damp and hold &kneeiii_leg stop &kneeiv_stance preparation/7(VceRF), negative half/1, negative half1/1  "VceRF"
  VceHAM/1 -> kneeii_damp and hold &kneeiii_leg stop &kneeiv_stance preparation/4(VceHAM), negative half2/1
  " 2"/1 -> Sum6/1  "HFL"
  " 3"/1 -> Sum6/2
  Sum6/1 -> Mux2/1  "HFL"
  negative half1/1 -> " 3"/1
  negative half2/1 -> " 6"/1
  " 5"/1 -> Sum7/1  "GLU"
  Sum7/1 -> Mux2/2  "GLU"
  " 6"/1 -> Sum7/2
  Constant4/1 -> Sum13/2
  Constant7/1 -> Sum2/2
  Constant6/1 -> Sum4/2
  Constant8/1 -> Sum10/1
  Sum10/1 -> Sum1/1  "lceOffRF"
  Sum4/1 -> " 4"/1
  Constant11/1 -> Sum14/2  "phi2lopt_BFSH"
  Constant14/1 -> Mux/4
  Constant12/1 -> Mux/2
  Mux/1 -> Prestimulations/1
  Constant19/1 -> Mux/9
  Constant17/1 -> Mux/6
  Constant18/1 -> Mux/7
  Constant15/1 -> Mux/1
  Constant13/1 -> Mux/3
  Constant16/1 -> Mux/5
  Constant20/1 -> Mux/8

== system NeuroMuscularLibrary/Swing Phase G&H ==
  note: Hip Torque
  note: Torques
  note: Stimulation
  note: GLU Control
  note: HFL Control
  note: GAS Control
  note: VAS Control
  note: TA Control
  note: SOL Control
  note: HAM Control
  Muscle Torques : Inport
  FmSOL : Inport  Port=2
  LceTA : Inport  Port=3
  FmHAM : Inport  Port=4
  FmGLU : Inport  Port=5
  LceHFL : Inport  Port=6
  LceHAM : Inport  Port=7
  phiANDdphiHAT : Inport  Port=8
  Add2 : Sum
  Add4 : Sum  Inputs=++-+
  Add7 : Sum
  Add8 : Sum
  Count Extend : dspswit3/Counter  Direction=Up  CountEvent=Rising edge  CounterSize=16 bits  MaxCount=255  InitialCount=0  Output=Count  HitValue=32  ResetInput=off  SamplesPerFrame=1  Ts=1  CntDtype=double  HitDtype=Logical
  Count Flex : dspswit3/Counter  Direction=Up  CountEvent=Rising edge  CounterSize=16 bits  MaxCount=255  InitialCount=0  Output=Count  HitValue=32  ResetInput=off  SamplesPerFrame=1  Ts=1  CntDtype=double  HitDtype=Logical
  Count Hold : dspswit3/Counter  Direction=Up  CountEvent=Rising edge  CounterSize=16 bits  MaxCount=255  InitialCount=0  Output=Count  HitValue=32  ResetInput=off  SamplesPerFrame=1  Ts=1  CntDtype=double  HitDtype=Logical
  Count Stancea : dspswit3/Counter  Direction=Up  CountEvent=Rising edge  CounterSize=16 bits  MaxCount=255  InitialCount=0  Output=Count  HitValue=32  ResetInput=off  SamplesPerFrame=1  Ts=1  CntDtype=double  HitDtype=Logical
  Count Stop : dspswit3/Counter  Direction=Up  CountEvent=Rising edge  CounterSize=16 bits  MaxCount=255  InitialCount=0  Output=Count  HitValue=32  ResetInput=off  SamplesPerFrame=1  Ts=1  CntDtype=double  HitDtype=Logical
  Demux : Demux  Outputs=3
  Demux2 : Demux  Outputs=2
  FB Gain1 : Gain  Gain=GainHAM  SaturateOnIntegerOverflow=on  OutDataTypeStr=Inherit: Same as input  ParamDataTypeStr=Inherit: Same as input
  FB Gain11 : Gain  Gain=Klean  SaturateOnIntegerOverflow=on  OutDataTypeStr=Inherit: Same as input  ParamDataTypeStr=Inherit: Same as input
  FB Gain2 : Gain  Gain=GainHFL  SaturateOnIntegerOverflow=on  OutDataTypeStr=Inherit: Same as input  ParamDataTypeStr=Inherit: Same as input
  FB Gain4 : Gain  Gain=GainHAMHFL  SaturateOnIntegerOverflow=on  OutDataTypeStr=Inherit: Same as input  ParamDataTypeStr=Inherit: Same as input
  FB Gain5 : Gain  Gain=GainGLU  SaturateOnIntegerOverflow=on  OutDataTypeStr=Inherit: Same as input  ParamDataTypeStr=Inherit: Same as input
  FB Gain8 : Gain  Gain=GainTA  SaturateOnIntegerOverflow=on  OutDataTypeStr=Inherit: Same as input  ParamDataTypeStr=Inherit: Same as input
  Mux2 : Mux  Inputs=3
  Mux3 : Mux  Inputs=5
  Mux4 : Mux  Inputs=3
  Mux5 : Mux  Inputs=7
  Stimulation Bias : Constant  Value=PreStimVAS
  Stimulation Bias1 : Constant  Value=PreStimGAS
  Stimulation Bias2 : Constant  Value=PreStimTA
  Stimulation Bias3 : Constant  Value=PreStimSOL
  Stimulation Bias4 : Constant  Value=PreStimHFL
  Stimulation Bias5 : Constant  Value=PreStimHAM
  Stimulation Bias6 : Constant  Value=phiHATref
  Stimulation Bias8 : Constant  Value=PreStimGLU
  Sum9 : Sum  Inputs=|+-  SaturateOnIntegerOverflow=on  InputSameDT=on  OutDataTypeStr=Inherit: Same as first input
  Terminator : Terminator
  Terminator1 : Terminator
  ideal ankle torque{,1..7} (8 alike) : Constant  Value=0
  Stimulation : Outport
  Swing Ideal Torques : Outport  Port=2
  Swing Muscle Torques : Outport  Port=3
  Swing State Counts : Outport  Port=4
  wires:
  Count Extend/1 -> Mux3/5
  Count Stop/1 -> Mux3/4
  Count Hold/1 -> Mux3/3
  Count Flex/1 -> Mux3/2
  Mux3/1 -> Swing State Counts/1
  Count Stancea/1 -> Mux3/1
  ideal ankle torque/1 -> Mux2/3
  Mux2/1 -> Swing Ideal Torques/1
  Mux4/1 -> Swing Muscle Torques/1
  Muscle Torques/1 -> Demux/1
  Demux/1 -> Mux4/1
  Demux/2 -> Mux4/2
  Demux/3 -> Mux4/3
  Stimulation Bias5/1 -> Add7/1
  Stimulation Bias1/1 -> Mux5/3
  FB Gain1/1 -> Add7/2
  Stimulation Bias/1 -> Mux5/4
  Mux5/1 -> Stimulation/1
  phiANDdphiHAT/1 -> Demux2/1
  Add8/1 -> Mux5/6
  Stimulation Bias2/1 -> Add2/2
  Demux2/1 -> Sum9/1  "phiHAT"
  Stimulation Bias8/1 -> Add8/1
  FB Gain5/1 -> Add8/2
  LceTA/1 -> FB Gain8/1
  Add7/1 -> Mux5/5
  Stimulation Bias6/1 -> Sum9/2
  Sum9/1 -> FB Gain11/1
  Add4/1 -> Mux5/7
  FmGLU/1 -> FB Gain5/1
  FmHAM/1 -> FB Gain1/1
  FB Gain8/1 -> Add2/1
  Stimulation Bias3/1 -> Mux5/1
  Add2/1 -> Mux5/2
  LceHFL/1 -> FB Gain2/1
  Stimulation Bias4/1 -> Add4/1
  FB Gain2/1 -> Add4/2
  LceHAM/1 -> FB Gain4/1
  FB Gain4/1 -> Add4/3
  Demux2/2 -> Terminator/1  "dphiHat"
  FB Gain11/1 -> Add4/4
  ideal ankle torque2/1 -> Mux2/1
  ideal ankle torque1/1 -> Mux2/2
  ideal ankle torque3/1 -> Count Stancea/1
  ideal ankle torque7/1 -> Count Extend/1
  ideal ankle torque6/1 -> Count Stop/1
  ideal ankle torque5/1 -> Count Hold/1
  ideal ankle torque4/1 -> Count Flex/1
  FmSOL/1 -> Terminator1/1

== system NeuroMuscularLibrary/Swing Phase Hip muscle ==
  note: only ankle muscle torque
  note: Hip Torque
  note: Torques
  note: VAS Control
  note: TA Control
  note: GAS Control
  note: SOL Control
  note: Stimulation
  note: GLU Control
  note: HAM Control
  note: HFL Control
  Muscle Torques : Inport
  LceTA : Inport  Port=2
  Leg Angle : Inport  Port=3
  Leg Length : Inport  Port=4
  Stance? : Inport  Port=5
  contraStance? : Inport  Port=6
  Knee Speed : Inport  Port=7
  Target Leg Angle : Inport  Port=8
  FmHAM : Inport  Port=9
  FmGLU : Inport  Port=10
  LceHFL : Inport  Port=11
  LceHAM : Inport  Port=12
  phiANDdphiHAT : Inport  Port=13
  " 1" : Gain  Gain=hipPGain
  " 2" : Gain  Gain=hipDGain
  " 3" : Gain  Gain=GainTA
  " 4" : Gain  Gain=2
  " 5" : Gain  Gain=0
  " 6" : Gain  Gain=0
  " 7" : Gain  Gain=0
  Add : Sum  Inputs=+++
  Add1 : Sum  Inputs=+-+
  Add3 : Sum
  Add4 : Sum  Inputs=++-+
  Add7 : Sum
  Add8 : Sum
  Chart : Stateflow chart  TreatAsAtomicUnit=on
  Constant1 : Constant  Value=0
  Constant4 : Constant  Value=PreStimTA
  Constant5 : Constant  Value=0
  Constant6 : Constant  Value=0
  Count Extend : dspswit3/Counter  Direction=Up  CountEvent=Rising edge  CounterSize=16 bits  MaxCount=255  InitialCount=0  Output=Count  HitValue=32  ResetInput=off  SamplesPerFrame=1  Ts=1  CntDtype=double  HitDtype=Logical
  Count Flex : dspswit3/Counter  Direction=Up  CountEvent=Rising edge  CounterSize=16 bits  MaxCount=255  InitialCount=0  Output=Count  HitValue=32  ResetInput=off  SamplesPerFrame=1  Ts=1  CntDtype=double  HitDtype=Logical
  Count Hold : dspswit3/Counter  Direction=Up  CountEvent=Rising edge  CounterSize=16 bits  MaxCount=255  InitialCount=0  Output=Count  HitValue=32  ResetInput=off  SamplesPerFrame=1  Ts=1  CntDtype=double  HitDtype=Logical
  Count Stancea : dspswit3/Counter  Direction=Up  CountEvent=Rising edge  CounterSize=16 bits  MaxCount=255  InitialCount=0  Output=Count  HitValue=32  ResetInput=off  SamplesPerFrame=1  Ts=1  CntDtype=double  HitDtype=Logical
  Count Stop : dspswit3/Counter  Direction=Up  CountEvent=Rising edge  CounterSize=16 bits  MaxCount=255  InitialCount=0  Output=Count  HitValue=32  ResetInput=off  SamplesPerFrame=1  Ts=1  CntDtype=double  HitDtype=Logical
  Demux : Demux  Outputs=3
  Demux2 : Demux  Outputs=2
  FB Gain1 : Gain  Gain=GainHAM  SaturateOnIntegerOverflow=on  OutDataTypeStr=Inherit: Same as input  ParamDataTypeStr=Inherit: Same as input
  FB Gain11 : Gain  Gain=Klean  SaturateOnIntegerOverflow=on  OutDataTypeStr=Inherit: Same as input  ParamDataTypeStr=Inherit: Same as input
  FB Gain2 : Gain  Gain=GainHFL  SaturateOnIntegerOverflow=on  OutDataTypeStr=Inherit: Same as input  ParamDataTypeStr=Inherit: Same as input
  FB Gain4 : Gain  Gain=GainHAMHFL  SaturateOnIntegerOverflow=on  OutDataTypeStr=Inherit: Same as input  ParamDataTypeStr=Inherit: Same as input
  FB Gain5 : Gain  Gain=GainGLU  SaturateOnIntegerOverflow=on  OutDataTypeStr=Inherit: Same as input  ParamDataTypeStr=Inherit: Same as input
  Filtered Derivative : Subsystem
  Knee Flex : Subsystem  TreatAsAtomicUnit=on
  Knee Hold : Subsystem  TreatAsAtomicUnit=on
  Knee Stop : Subsystem  TreatAsAtomicUnit=on
  Multiply : Gain
  Multiply1 : Gain
  Multiply2 : Gain
  Mux1 : Mux  Inputs=7
  Mux2 : Mux  Inputs=3
  Mux3 : Mux  Inputs=5
  Mux4 : Mux  Inputs=3
  Stimulation Bias4 : Constant  Value=PreStimHFL
  Stimulation Bias5 : Constant  Value=PreStimHAM
  Stimulation Bias6 : Constant  Value=phiHATref
  Stimulation Bias8 : Constant  Value=PreStimGLU
  Sum : Sum  Inputs=|+-
  Sum9 : Sum  Inputs=|+-  SaturateOnIntegerOverflow=on  InputSameDT=on  OutDataTypeStr=Inherit: Same as first input
  Terminator : Terminator
  Wait 100 ms to enable : Subsystem
  Zero-Order Hold : ZeroOrderHold  SampleTime=.01
  ideal ankle torque : Constant  Value=0
  Stimulation : Outport
  Swing Ideal Torques : Outport  Port=2
  Swing Muscle Torques : Outport  Port=3
  Swing State Counts : Outport  Port=4
  wires:
  Wait 100 ms to enable/1(Out1) -> Chart/4(legAngleSpeed), Knee Hold/1(legAngleSpeed), Knee Stop/1(legAngleSpeed), Knee Flex/1(LegAngleSpeed), " 2"/1
  Filtered Derivative/1(Out1) -> Wait 100 ms to enable/1(In1)
  Target Leg Angle/1 -> Sum/1, Chart/5(legAngleTgt), Knee Stop/3(legAngleTgt), Knee Hold/3(legAngleTgt)
  " 2"/1 -> Add1/2
  " 1"/1 -> Add1/1
  Sum/1 -> " 1"/1
  Leg Angle/1 -> Filtered Derivative/1(In1), Chart/3(legAngle), Knee Stop/2(legAngle), Knee Hold/2(legAngle), Sum/2  "Leg Angle"
  Mux1/1 -> Stimulation/1
  Add4/1 -> Mux1/7
  Add8/1 -> Mux1/6
  Add7/1 -> Mux1/5
  Constant1/1 -> Mux1/4
  Constant5/1 -> Mux1/3
  Constant6/1 -> Mux1/1
  Add3/1 -> Mux1/2
  LceTA/1 -> " 3"/1
  " 3"/1 -> Add3/2
  Constant4/1 -> Add3/1
  Knee Speed/1 -> Knee Hold/4(kneeSpeed)
  Knee Hold/1(tau) -> Add/2
  Knee Flex/1(tau) -> Add/1
  Knee Stop/1(tau) -> " 4"/1, Add/3
  Add/1 -> Mux2/2
  " 4"/1 -> Add1/3
  Chart/1(flex) -> Knee Flex/Enable, Count Flex/1
  Chart/2(hold) -> Count Hold/1, Knee Hold/Enable
  Chart/3(stop) -> Count Stop/1, Knee Stop/Enable
  Chart/4(extend) -> Count Extend/1, Knee Stop/5(Extend?)
  Stance?/1 -> Zero-Order Hold/1, Chart/1(Stance)
  contraStance?/1 -> Chart/2(contraStance)
  Leg Length/1 -> Chart/6(legLength), Knee Stop/4(Leg Length)
  Add1/1 -> " 7"/1  "Hip Torque"
  Count Extend/1 -> Mux3/5
  Count Stop/1 -> Mux3/4
  Count Hold/1 -> Mux3/3
  Count Flex/1 -> Mux3/2
  Mux3/1 -> Swing State Counts/1
  Count Stancea/1 -> Mux3/1
  Zero-Order Hold/1 -> Count Stancea/1
  ideal ankle torque/1 -> Mux2/3
  Mux2/1 -> Swing Ideal Torques/1
  Mux4/1 -> Swing Muscle Torques/1
  Muscle Torques/1 -> Demux/1
  Demux/1 -> " 5"/1
  Demux/2 -> " 6"/1
  " 5"/1 -> Mux4/1
  " 6"/1 -> Mux4/2
  Demux/3 -> Mux4/3
  FB Gain1/1 -> Add7/2
  Multiply/1 -> Add8/1
  FB Gain5/1 -> Add8/2
  FB Gain11/1 -> Add4/4
  Multiply1/1 -> Add4/1
  Demux2/2 -> Terminator/1  "dphiHat"
  FB Gain4/1 -> Add4/3
  Stimulation Bias4/1 -> Multiply1/1
  FB Gain2/1 -> Add4/2
  LceHAM/1 -> FB Gain4/1
  FmHAM/1 -> FB Gain1/1
  Stimulation Bias6/1 -> Sum9/2
  Stimulation Bias8/1 -> Multiply/1
  Sum9/1 -> FB Gain11/1
  phiANDdphiHAT/1 -> Demux2/1
  FmGLU/1 -> FB Gain5/1
  Demux2/1 -> Sum9/1  "phiHAT"
  LceHFL/1 -> FB Gain2/1
  Multiply2/1 -> Add7/1
  Stimulation Bias5/1 -> Multiply2/1
  " 7"/1 -> Mux2/1
